simulink model "MotorSoftStart"  (R2025a)
settings: Solver=VariableStepAuto  StartTime=0.0  StopTime=10.0  RelTol=1e-3
settings Model: Creator=mahij  LastModifiedBy=mahij

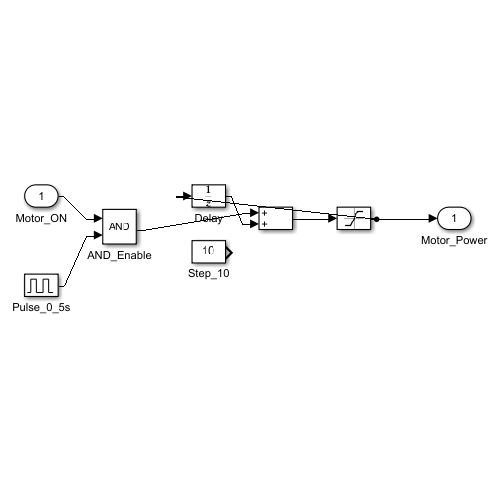
[thumbnail: Simulink's stored preview of the top-level diagram]
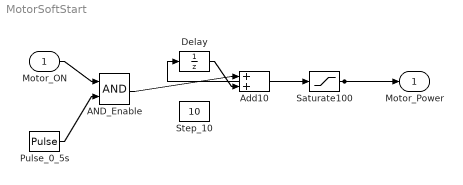
== system MotorSoftStart ==
  Motor_ON : Inport
  AND_Enable : Logic  AllPortsSameDT=off  OutDataTypeStr=boolean
  Add10 : Sum
  Delay : UnitDelay  SampleTime=0.5  HasFrameUpgradeWarning=on
  Pulse_0_5s : DiscretePulseGenerator  PulseType=Time based  Period=1  PulseWidth=50  SampleTime=0.5
  Saturate100 : Saturate  UpperLimit=100  LowerLimit=0
  Step_10 : Constant  Value=10
  Motor_Power : Outport
  wires:
  Motor_ON/1 -> AND_Enable/1
  Pulse_0_5s/1 -> AND_Enable/2
  AND_Enable/1 -> Add10/1
  Delay/1 -> Add10/2
  Add10/1 -> Saturate100/1
  Saturate100/1 -> Motor_Power/1, Delay/1
